simulink model "IP_LQG_MIO16E4_2015a"  (R2015a)
settings: Solver=ode3  StartTime=0.0  StopTime=200  RelTol=1e-3
values from neighbouring files (symbols this model uses):
  A = [A zeros(5,1) ... (first row only)    [IP_MACRO_Int.m]    (also in IP_MACRO_Int_BEST.m; Integrador.mat = [0 0 0 0 0 1 1 -0.0174048595758 0 -0.0173759205618 -232.0252; Q_100_10_10_0_0__R_0_25.mat = [0 0 0 0 0 1 -0.0174048595758 0 -0.0173759205618 -232.025201; Q_100_10_1_0_0__R_0_1__Perturbacao.mat = [0 0 0 0 0 1 -0.0174048595758 0 -0.0173759205618 -232.025201)
  ALPHA_MAX = 90 * pi/180    (= 1.57079632679)    [IP_MACRO_Int.m]    (also in IP_MACRO_Int_BEST.m; Integrador.mat; Q_100_10_10_0_0__R_0_25.mat; Q_100_10_1_0_0__R_0_1__Perturbacao.mat)
  B = [B; 0]    [IP_MACRO_Int.m]    (also in IP_MACRO_Int_BEST.m; Integrador.mat = [0 0 0 0 333.33674813 0]; Q_100_10_10_0_0__R_0_25.mat = [0 0 0 0 333.33674813]; Q_100_10_1_0_0__R_0_1__Perturbacao.mat = [0 0 0 0 333.33674813])
  BETA_MAX = 15 * pi/180    (= 0.261799387799)    [IP_MACRO_Int.m]    (also in IP_MACRO_Int_BEST.m; Integrador.mat; Q_100_10_10_0_0__R_0_25.mat; Q_100_10_1_0_0__R_0_1__Perturbacao.mat)
  C = [1 0 0 0 0 0 ... (first row only)    [IP_MACRO_Int.m]    (also in IP_MACRO_Int_BEST.m; Integrador.mat = [1 0 0 0 0 0 0 1 0 0 0 0 ... (18 elements, 3x6)]; Q_100_10_10_0_0__R_0_25.mat = [1  0  0  0  0; 0  0  1  0  0]; Q_100_10_1_0_0__R_0_1__Perturbacao.mat = [1  0  0  0  0; 0  0  1  0  0])
  K = lqr(A, B, Qr, Rr)    [IP_MACRO_Int.m]    (also in IP_MACRO_Int_BEST.m; Integrador.mat = [-31.6290452542 -20.522155178 202.844137505 30.7284869207 0.; Q_100_10_10_0_0__R_0_25.mat = [-19.9999999997 -13.3101285986 130.968964914 19.7745514964 0; Q_100_10_1_0_0__R_0_1__Perturbacao.mat = [-31.6227765982 -20.5206927522 202.834413955 30.727005876 0.)
  L = lqe(A, G, C, Qe, Re)    [IP_MACRO_Int.m]    (also in IP_MACRO_Int_BEST.m; Integrador.mat = [3.22899659182 0.983246447527 1.1385177435 8.08815299126 -0.; Q_100_10_10_0_0__R_0_25.mat = [3.26664981927  1.13709483629; 0.981992854244  11.8725297148; Q_100_10_1_0_0__R_0_1__Perturbacao.mat = [3.26664981927  1.13709483629; 0.981992854244  11.8725297148)
  TIME_DELAY = 6    [IP_MACRO_Int.m]    (also in IP_MACRO_Int_BEST.m; Integrador.mat; Q_100_10_10_0_0__R_0_25.mat; Q_100_10_1_0_0__R_0_1__Perturbacao.mat)
  Ts = 0.001    [IP_MACRO_Int.m]    (also in IP_MACRO_Int_BEST.m; Integrador.mat; Q_100_10_10_0_0__R_0_25.mat; Q_100_10_1_0_0__R_0_1__Perturbacao.mat)
  V_MAX = 5    [IP_MACRO_Int.m]    (also in IP_MACRO_Int_BEST.m; Integrador.mat; Q_100_10_10_0_0__R_0_25.mat; Q_100_10_1_0_0__R_0_1__Perturbacao.mat)
  V_MIN = -5    [IP_MACRO_Int.m]    (also in IP_MACRO_Int_BEST.m; Integrador.mat; Q_100_10_10_0_0__R_0_25.mat; Q_100_10_1_0_0__R_0_1__Perturbacao.mat)
undefined symbols (not defined in the file or in its folder): MIO, National_Instruments, PCI
libraries: sldrtlib x3, simulink x2
settings Model: SimulationMode=external  ExtModeTrigDuration=100000  Creator=Alunos  LastModifiedBy=Alunos
settings HardwareCC: ProdIntDivRoundTo=Zero  ProdEndianess=LittleEndian  ProdHWDeviceType=Intel->x86/Pentium  TargetIntDivRoundTo=Zero  TargetEndianess=LittleEndian  TargetHWDeviceType=Intel->x86/Pentium
settings RTWCC: SystemTargetFile=rtwin.tlc  TemplateMakefile=rtwin.tmf  Description=Simulink Desktop Real-Time  RTWCompilerOptimization=on
settings CodeAppCC: MaxIdLength=95
settings RTWinTargetCC: TargetPreCompLibLocation=C:\Program Files\MATLAB\R2015a\toolbox\sldrt\lib\win32

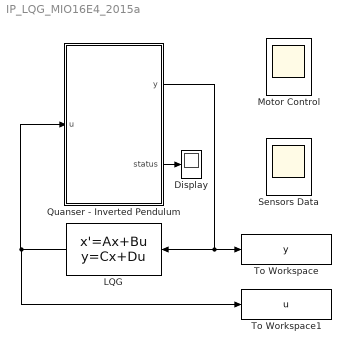
== system IP_LQG_MIO16E4_2015a ==
  Display : Display
  LQG : StateSpace  A=A-B*K-L*C  B=L  C=-K  D=zeros(1,2)  X0=0
  Motor Control : Scope
      settings: Floating=on  ShowLegends=on  SaveName=ScopeData2
  Quanser - Inverted Pendulum : Subsystem
      mask Display: image('IP_QUANSER.jpg');
  Sensors Data : Scope
      settings: Floating=on  ShowLegends=on  YMin=-3.191592653589793  YMax=3.191592653589793
  To Workspace : ToWorkspace  VariableName=y  SampleTime=-1
  To Workspace1 : ToWorkspace  VariableName=u  SampleTime=-1
  wires:
  Quanser - Inverted Pendulum/1(y) -> LQG/1, To Workspace/1
  LQG/1 -> To Workspace1/1, Quanser - Inverted Pendulum/1(u)
  Quanser - Inverted Pendulum/2(status) -> Display/1

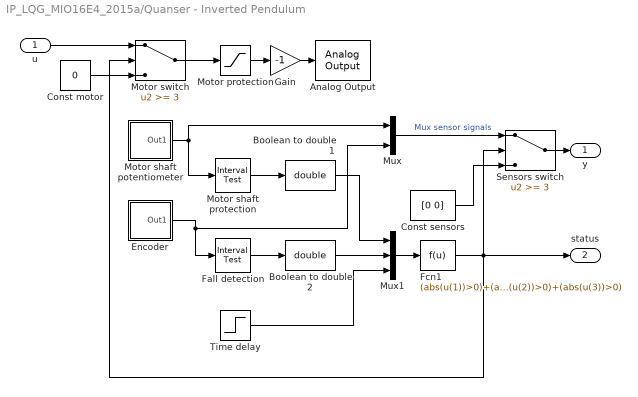
== system IP_LQG_MIO16E4_2015a/Quanser - Inverted Pendulum ==
  u : Inport
  Analog Output : sldrtlib/Analog Output  SampleTime=Ts  MaxMissedTicks=10  ShowMissedTicks=off  YieldWhenWaiting=off  DrvName=National_Instruments/PCI-MIO-16E-4  DrvAddress=4294967295  DrvOptions=[0 0 0 0 0 0]  Channels=1  RangeMode=1  VoltRange=1  InitialValue=0  FinalValue=0
      settings: AttributesFormatString=National Instruments\nPCI-MIO-16E-4 [auto]
  Boolean to double 1 : DataTypeConversion  OutDataTypeStr=double
  Boolean to double 2 : DataTypeConversion  OutDataTypeStr=double
  Const motor : Constant  Value=0
  Const sensors : Constant  Value=[0 0]
  Encoder : Subsystem
  Fall detection : simulink/Logic and Bit Operations/Interval Test  IntervalClosedRight=on  uplimit=BETA_MAX  IntervalClosedLeft=on  lowlimit=-BETA_MAX  OutDataTypeStr=uint8
  Fcn1 : Fcn  Expr=(abs(u(1))>0)+(abs(u(2))>0)+(abs(u(3))>0)
  Gain : Gain  Gain=-1
  Motor protection : Saturate  UpperLimit=V_MAX  LowerLimit=V_MIN
  Motor shaft potentiometer : Subsystem
  Motor shaft protection : simulink/Logic and Bit Operations/Interval Test  IntervalClosedRight=on  uplimit=ALPHA_MAX  IntervalClosedLeft=on  lowlimit=-ALPHA_MAX  OutDataTypeStr=uint8
  Motor switch : Switch  Threshold=3
  Mux : Mux  Inputs=2
  Mux1 : Mux  Inputs=3
  Sensors switch : Switch  Threshold=3
  Time delay : Step  Time=TIME_DELAY  SampleTime=0
  y : Outport
  status : Outport  Port=2
  wires:
  u/1 -> Motor switch/1
  Motor switch/1 -> Motor protection/1
  Const motor/1 -> Motor switch/3
  Motor shaft potentiometer/1(Out1) -> Mux/1, Motor shaft protection/1
  Encoder/1(Out1) -> Fall detection/1, Mux/2
  Mux1/1 -> Fcn1/1
  Time delay/1 -> Mux1/3
  Fall detection/1 -> Boolean to double 2/1
  Boolean to double 2/1 -> Mux1/2
  Motor shaft protection/1 -> Boolean to double 1/1
  Boolean to double 1/1 -> Mux1/1
  Const sensors/1 -> Sensors switch/3
  Mux/1 -> Sensors switch/1  "Mux sensor signals"
  Sensors switch/1 -> y/1
  Gain/1 -> Analog Output/1
  Motor protection/1 -> Gain/1
  Fcn1/1 -> status/1, Motor switch/2, Sensors switch/2

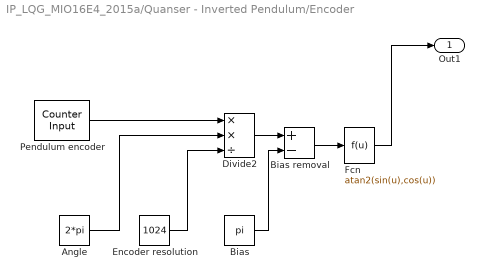
== system IP_LQG_MIO16E4_2015a/Quanser - Inverted Pendulum/Encoder ==
  Angle : Constant  Value=2*pi
  Bias : Constant  Value=pi
  Bias removal : Sum  Inputs=+-
  Divide2 : Product  Inputs=**/
  Encoder resolution : Constant  Value=1024
  Fcn : Fcn  Expr=atan2(sin(u),cos(u))
  Pendulum encoder : sldrtlib/Counter Input  SampleTime=Ts  MaxMissedTicks=10  ShowMissedTicks=off  YieldWhenWaiting=off  DrvName=National_Instruments/PCI-MIO-16E-4  DrvAddress=4294967295  DrvOptions=[0 0 0 0 1 0]  Channels=2  ResetMode=1  CounterEdge=1  CounterGate=1  DataType=1
      settings: AttributesFormatString=National Instruments\nPCI-MIO-16E-4 [auto]
  Out1 : Outport
  wires:
  Bias/1 -> Bias removal/2
  Encoder resolution/1 -> Divide2/3
  Divide2/1 -> Bias removal/1
  Fcn/1 -> Out1/1
  Pendulum encoder/1 -> Divide2/1
  Bias removal/1 -> Fcn/1
  Angle/1 -> Divide2/2

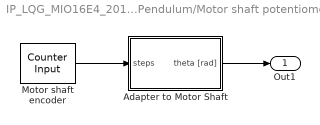
== system IP_LQG_MIO16E4_2015a/Quanser - Inverted Pendulum/Motor shaft potentiometer ==
  Adapter to Motor Shaft : Subsystem
  Motor shaft encoder : sldrtlib/Counter Input  SampleTime=Ts  MaxMissedTicks=10  ShowMissedTicks=off  YieldWhenWaiting=off  DrvName=National_Instruments/PCI-MIO-16E-4  DrvAddress=4294967295  DrvOptions=[0 0 0 0 1 0]  Channels=1  ResetMode=1  CounterEdge=1  CounterGate=1  DataType=1
      settings: AttributesFormatString=National Instruments\nPCI-MIO-16E-4 [auto]
  Out1 : Outport
  wires:
  Motor shaft encoder/1 -> Adapter to Motor Shaft/1(steps)
  Adapter to Motor Shaft/1(theta [rad]) -> Out1/1

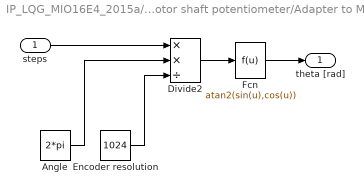
== system IP_LQG_MIO16E4_2015a/Quanser - Inverted Pendulum/Motor shaft potentiometer/Adapter to Motor Shaft ==
  steps : Inport
  Angle : Constant  Value=2*pi
  Divide2 : Product  Inputs=**/
  Encoder resolution : Constant  Value=1024
  Fcn : Fcn  Expr=atan2(sin(u),cos(u))
  theta [rad] : Outport
  wires:
  Angle/1 -> Divide2/2
  Encoder resolution/1 -> Divide2/3
  steps/1 -> Divide2/1
  Divide2/1 -> Fcn/1
  Fcn/1 -> theta [rad]/1
